simulink subsystem "CasADi_freetf_delay"  (R2024b)
settings: Solver=VariableStepAuto  StartTime=0.0  StopTime=10.0  RelTol=1e-3
settings Model: Creator=thatf  LastModifiedBy=thatf

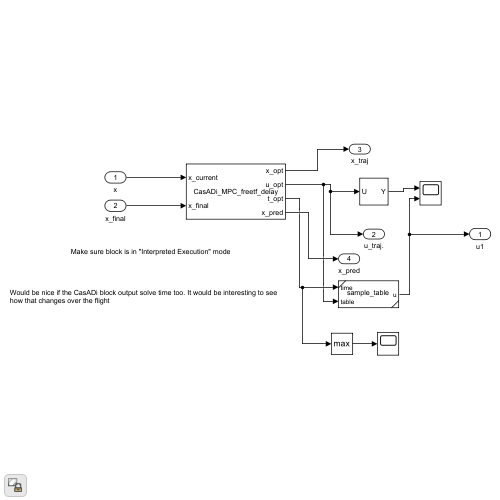
[thumbnail: Simulink's stored preview of the top-level diagram]
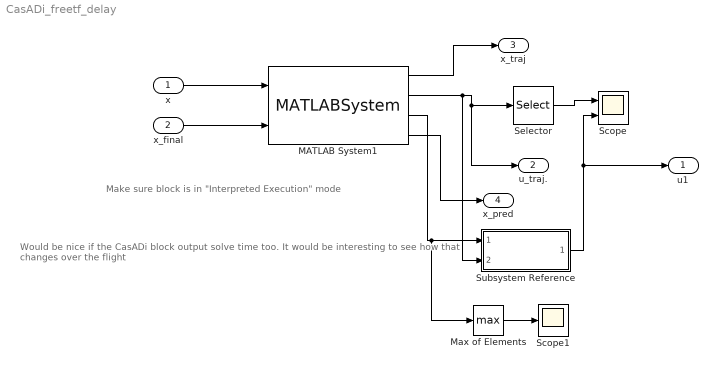
== system CasADi_freetf_delay ==
  note: Make sure block is in "Interpreted Execution" mode
  note: Would be nice if the CasADi block output solve time too. It would be interesting to see how that changes over the flight
  x : Inport
  x_final : Inport  Port=2
  MATLAB System1 : MATLABSystem  System=CasADi_MPC_freetf_delay  vehicle=vehicle  max_t_step=0.5  steps=steps  max_iter=max_iter  x_initial=x0  x_final=xf  delay_time=optimization_time  SimulateUsing=Interpreted execution
      mask Type: CasADi_MPC_freetf_delay
      mask Display:
      | disp('CasADi_MPC_freetf_delay');
      | port_label('input',1,'x_current');
      | port_label('input',2,'x_final');
      | port_label('output',1,'x_opt');
      | port_label('output',2,'u_opt');
      | port_label('output',3,'t_opt');
      | port_label('output',4,'x_pred');
  Max of Elements : MinMax  Function=max
  Scope : Scope  NumInputPorts=2
  Scope1 : Scope
  Selector : Selector  NumberOfDimensions=2  InputPortWidth=3  IndexOptions=Index vector (dialog),Select all  Indices=[1],1  OutputSizes=1,1
  Subsystem Reference : Subsystem  ReferencedSubsystem=sample_table
  u1 : Outport
  u_traj. : Outport  Port=2
  x_traj : Outport  Port=3
  x_pred : Outport  Port=4
  wires:
  Selector/1 -> Scope/1
  x/1 -> MATLAB System1/1
  MATLAB System1/1 -> x_traj/1
  MATLAB System1/2 -> Subsystem Reference/2, u_traj./1, Selector/1
  MATLAB System1/4 -> x_pred/1
  MATLAB System1/3 -> Subsystem Reference/1, Max of Elements/1
  Subsystem Reference/1 -> u1/1, Scope/2
  x_final/1 -> MATLAB System1/2
  Max of Elements/1 -> Scope1/1
